simulink model "Hexa_CAD_ANSFT_Sim_V3"  (R2023a)
settings: Solver=ode4  StartTime=0.0  StopTime=30  FixedStep=0.01  RelTol=1e-3
model workspace (MAT data in the model file):
  hover_2m = [0 0 2 0 0 0 0 0 2 0 0 0 ... (36 elements, 6x6)]
  square = [0 0 2.5 0 0 0 0 0 2.5 0 0 0 ... (36 elements, 6x6)]
  tf : Simulink.Parameter (value not decoded)
  tray0 = [0 0 0 0 0 0 0.2 0.15 2 0 0 0 ... (36 elements, 6x6)]
  tray1 = [0 0 0 0 0 0 0 0 2 0 0 0 ... (36 elements, 6x6)]
  tray2 = [0 0 0 0 0 0 2 0 5 0 0 0 ... (36 elements, 6x6)]
  tray3 = [0 0 0 0 0 0 2 0 5 0 0 0 ... (36 elements, 6x6)]
  tray4 = [0 0 0 0 0 0 2 0 5 0.15 0 0 ... (36 elements, 6x6)]
  tray5 = [0 0 0 0 0 0 0 0 5 0.15 0 0 ... (36 elements, 6x6)]
  tray_yaw = [0 0 0 0 0 0 0 0 5 0 0 0 ... (36 elements, 6x6)]
undefined symbols (not defined in the file or in its folder): F, Light, MIL, smiData, X, Y, Z
libraries: sm_lib x168, nesl_utility x33, dspsrcs4 x9, sharedtransform x3, simulink x3, robotcorelib x1, aerolibwind2 x1
(part 3 of 6)

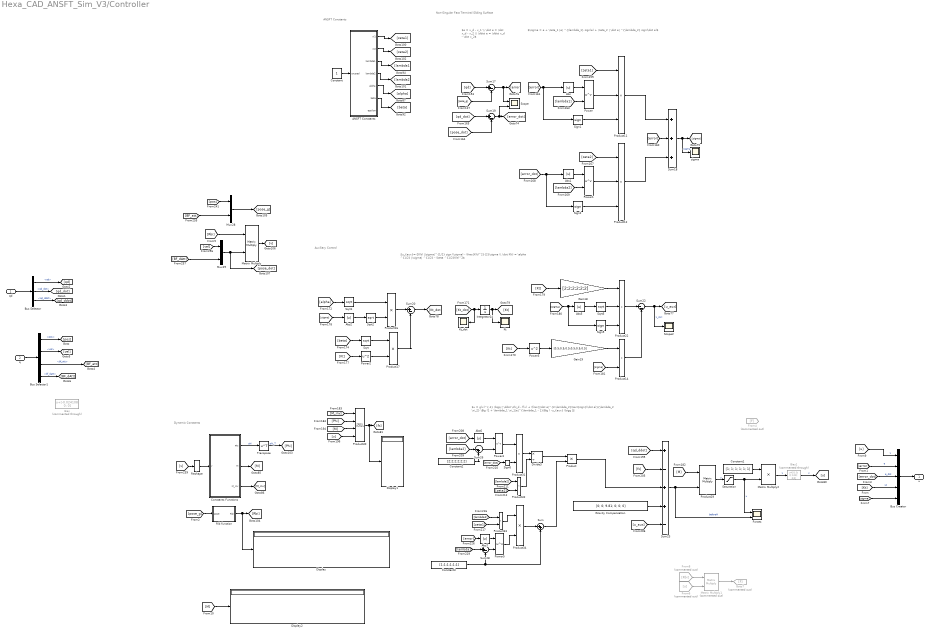
== system Hexa_CAD_ANSFT_Sim_V3/Controller ==
  note: $u = g(x)^{-1} \bigg [ \ddot \chi_d - f(x) + \frac{|\dot e|^{2-\lambda_2}\text{sign}(\dot e)}{\lambda_2 \xi_2} \Big (1 + \lambda_1 \xi_1|e|^{\lambda_1 - 1}\Big ) -u_{aux} \bigg ]$
  note: $e = x_d - x_1 \\ \dot e = \dot x_d - x_2 \\ \ddot e = \ddot x_d - \dot x_2$
  note: Non-Singular Fast Terminal Sliding Surface
  note: $\sigma = e + \zeta_1 |e| ^{\lambda_1} sign(e) + \zeta_2 | \dot e| ^{\lambda_2} sign(\dot e)$
  note: $u_{aux}=-2K(t) |\sigma|^{1/2} sign (\sigma) - \frac{K(t)^2}{2}\sigma \\ \dot K(t) = \alpha ^{1/2} |\sigma| ^{1/2} - \beta ^{1/2}K(t)^2$
  note: Auxiliary Control
  note: ANSFT Constants
  note: Dynamic Constants
  qd : Inport
  q : Inport  Port=2
  ANSFT Constants : MATLAB Function  TreatAsAtomicUnit=on
  Abs{,1..2,5..7} (6 alike) : Abs  SaturateOnIntegerOverflow=off
  Bias : Bias  Commented=through  Bias=[-0.024108; 0; 0]  SaturateOnIntegerOverflow=off
  Bias1 : Bias  Commented=through  Bias=[0; 0; 0; 0.02; 0;0]  SaturateOnIntegerOverflow=off
  Bus Creator : BusCreator  Inputs=5
  Bus Selector : BusSelector  OutputSignals=qd,qd_dot,qd_ddot
  Bus Selector1 : BusSelector  OutputSignals=pos,vel,bf_att,bf_datt
  Constant : Constant
  Constant1 : Constant  Value=[1; 1; 1; 1; 1; 1]
  Constant2 : Constant  Value=[2;2;2;2;2;2]
  Constant3 : Constant  Value=[1;1;1;1;1;1]
  Constants Functions : MATLAB Function  TreatAsAtomicUnit=on
  Display : Display
  Display1 : Display
  Display2 : Display
  Divide3 : Product  Inputs=*/
  Forces : Scope  NumInputPorts=2
  From4 : From  Commented=on  GotoTag=F
  From6 : From  Commented=on  GotoTag=u
  From8 : From  Commented=on  GotoTag=Rbi
  Gain18 : Gain  Gain=[2;2;2;2;2;2]
  Gain19 : Gain  Gain=[0.5;0.5;0.5;0.5;0.5;0.5]
  Goto7 : Goto  Commented=on  GotoTag=F
  Gravity Compensation : Constant  Value=[0; 0; 9.81; 0; 0; 0]
  Integrator14 : Integrator  InitialCondition=[0;0;0;0;0;0]
  Kt : Scope
  Kt_dot : Scope
  Matrix Multiply : Product  Multiplication=Matrix(*)
  Matrix Multiply1 : Product  Commented=on  Multiplication=Matrix(*)
  Matrix Multiply2 : Product
  Mux28 : Mux  Inputs=2
  Mux29 : Mux  Inputs=2
  Power{,1,4..5} (4 alike) : Math  Operator=pow
  Power2 : Math  Operator=square
  Power3 : Math  Operator=square
  Product{,14,16..17,31..34} (8 alike) : Product
  Product11 : Product  Inputs=3
  Product12 : Product  Inputs=3
  Product22 : Product  Inputs=3
  Product29 : Product  Multiplication=Matrix(*)
  Product30 : Product  Inputs=4  Multiplication=Matrix(*)
  Reshape : Reshape  OutputDimensionality=Customize  OutputDimensions=[6,1]
  Rib function : MATLAB Function  TreatAsAtomicUnit=on
  Saturation : Saturate  UpperLimit=[5; 5; 35; 0.2; 0.2; 0.2]  LowerLimit=[-5; -5; 0; -0.2; -0.2; -0.2]
  Scope : Scope  NumInputPorts=2
  Scope2 : Scope
  Sign{1..2,5..6} (4 alike) : Signum
  Sqrt{,1..2,5} (4 alike) : Sqrt
  Sum : Sum  Inputs=|++
  Sum{17,19..20,28} (4 alike) : Sum  Inputs=|+-
  Sum18 : Sum  Inputs=+++
  Sum22 : Sum  Inputs=|--
  Sum23 : Sum  Inputs=+-++-
  Sum26 : Sum  Inputs=|-+
  Transpose : Math  Operator=transpose
  sigma : Scope
  u : Outport
  wires:
  [zeta2] -> Product12/1
  [lambda1] -> Power/2
  Abs1/1 -> Power1/1
  [Kt] -> Power3/1
  [pose_g] -> Sum17/2
  Power5/1 -> Product34/2
  ANSFT Constants/4(lambda2) -> [lambda2]
  [Phi] -> Product30/2
  Product17/1 -> Sum20/2
  [v] -> Product30/4
  Sum20/1 -> [Kt_dot]
  [zeta2] -> Product32/2
  Sum19/1 -> Scope/2, [error_dot]
  Power4/1 -> Product31/1
  [error] -> Abs7/1
  [M_inv] -> Product30/1
  Product11/1 -> Sum18/1
  [lambda2] -> Power1/2
  [error_dot] -> Sign6/1
  [u_aux] -> Sum23/5
  Gain19/1 -> Product14/1
  [Kt] -> Gain18/1
  Sign2/1 -> Product12/3
  Gravity Compensation/1 -> Sum23/4
  ANSFT Constants/6(beta) -> [beta]
  [lambda1] -> Sum28/1
  Product14/1 -> Sum22/2
  Sum28/1 -> Power5/2
  Gain18/1 -> Product22/1
  Product12/1 -> Sum18/3
  [alpha] -> Sqrt1/1
  Product/1 -> Sum23/3
  Power2/1 -> Product17/2
  [M] -> Product29/1
  [beta] -> Sqrt/1
  [sigma] -> Abs2/1
  [fx] -> Sum23/2
  ANSFT Constants/3(lambda1) -> [lambda1]
  [M] -> Product30/3
  Product16/1 -> Sum20/1
  [error_dot] -> Sign2/1, Abs1/1
  Sqrt1/1 -> Product16/1
  Sqrt/1 -> Product17/1
  Abs2/1 -> Sqrt2/1
  [lambda2] -> Sum26/1
  [zeta1] -> Product33/2
  Sign6/1 -> Product31/2
  [qd_ddot] -> Sum23/1
  [error_dot] -> Abs6/1
  [lambda2] -> Product32/1
  Sign5/1 -> Product22/3
  Constant3/1 -> Sum28/2, Sum/2
  [zeta1] -> Product11/1
  ANSFT Constants/1(xi1) -> [zeta1]
  [sigma] -> Sign5/1, Abs5/1
  [error] -> Sum18/2
  Abs7/1 -> Power5/1
  Sum17/1 -> Scope/1, [error]
  Power/1 -> Product11/2
  Constant2/1 -> Sum26/2
  [sigma] -> Product14/2
  ANSFT Constants/5(alpha) -> [alpha]
  [qd_dot] -> Sum19/1
  Product32/1 -> Divide3/2
  [pose_dot] -> Sum19/2
  Sum23/1 -> Forces/2, Product29/2  "beforeM"
  Sum22/1 -> Scope2/1, [u_aux]  "u_aux"
  Abs/1 -> Power/1
  Abs5/1 -> Sqrt5/1
  Product33/1 -> Product34/1
  Product31/1 -> Divide3/1
  [error] -> Sign1/1, Abs/1
  Integrator14/1 -> Kt/1, [Kt]
  [Kt_dot] -> Kt_dot/1, Integrator14/1
  Sqrt5/1 -> Product22/2
  Product22/1 -> Sum22/1
  [Kt] -> Power2/1
  Sum18/1 -> sigma/1, [sigma]  "sigma"
  Power1/1 -> Product12/2
  [qd] -> Sum17/1
  Abs6/1 -> Power4/1
  Sum26/1 -> Power4/2
  ANSFT Constants/2(xi2) -> [zeta2]
  Divide3/1 -> Product/1
  Sqrt2/1 -> Product16/2
  Product30/1 -> Display1/1, [fx]
  [lambda1] -> Product33/1
  Constant/1 -> ANSFT Constants/1(unused)
  Sign1/1 -> Product11/3
  Power3/1 -> Gain19/1
  qd/1 -> Bus Selector/1
  Bus Selector/2 -> [qd_dot]  "<qd_dot>"
  Bus Selector/1 -> [qd]  "<qd>"
  Bus Selector/3 -> [qd_ddot]  "<qd_ddot>"
  Reshape/1 -> Constants Functions/1(v)
  Constants Functions/1(Phi) -> Transpose/1  "phi"
  Constants Functions/2(M) -> [M]
  Rib function/1(Rbi) -> Display/1, [Rbi]
  [v] -> Reshape/1
  Constants Functions/3(M_inv) -> [M_inv]
  [pose_g] -> Rib function/1(pose)
  Transpose/1 -> [Phi]  "phi_T"
  Mux28/1 -> [pose_g]
  Mux29/1 -> [pose_dot], Matrix Multiply/2
  [BF_dAtt] -> Mux29/2
  Matrix Multiply/1 -> [v]
  [Rbi] -> Matrix Multiply/1
  [pos] -> Mux28/1
  [BF_att] -> Mux28/2
  [vel] -> Mux29/1
  Bus Creator/1 -> u/1
  [error_dot] -> Bus Creator/3  "e_dot"
  [sigma] -> Bus Creator/5
  [Kt] -> Bus Creator/4  "kt"
  [error] -> Bus Creator/2  "e"
  q/1 -> Bus Selector1/1
  Bus Selector1/1 -> [pos]  "<pos>"
  Bus Selector1/3 -> [BF_att]  "<bf_att>"
  Bus Selector1/2 -> [vel]  "<vel>"
  Bus Selector1/4 -> [BF_dAtt]  "<bf_datt>"
  Product34/1 -> Sum/1
  Sum/1 -> Product/2
  Product29/1 -> Saturation/1  "u"
  From6/1 -> Matrix Multiply1/2
  From8/1 -> Matrix Multiply1/1
  Matrix Multiply1/1 -> Goto7/1
  [u] -> Bus Creator/1  "u"
  Saturation/1 -> Matrix Multiply2/2, Forces/1  "u"
  [M] -> Display2/1
  Matrix Multiply2/1 -> Bias1/1  "u"
  Constant1/1 -> Matrix Multiply2/1
  Bias1/1 -> [u]  "u"

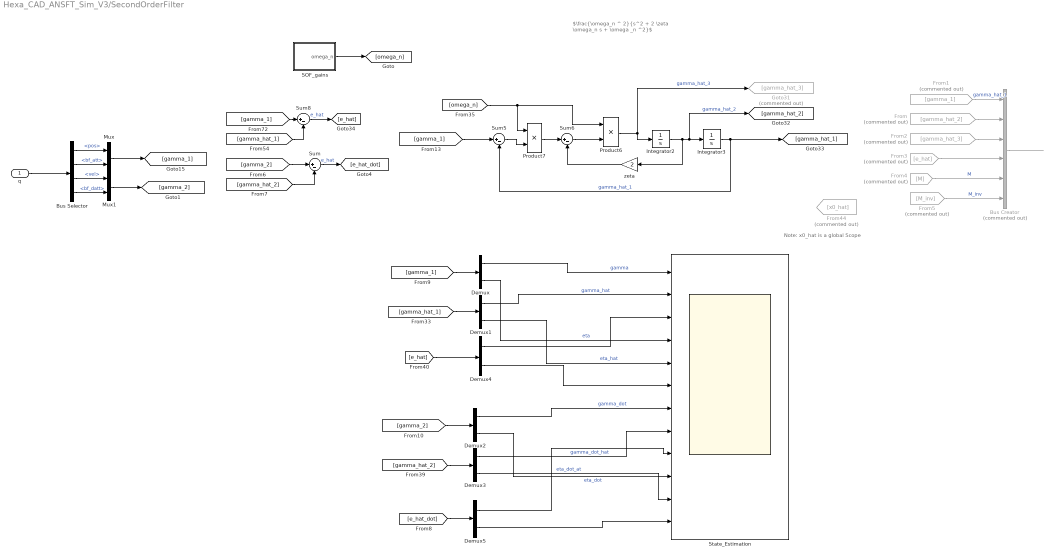
== system Hexa_CAD_ANSFT_Sim_V3/SecondOrderFilter ==
  note: Note: x0_hat is a global Scope
  note: $\frac{\omega_n ^ 2}{s^2 + 2 \zeta \omega_n s + \omega _n ^2}$
  q : Inport
  Bus Creator : BusCreator  Commented=on  Inputs=6
  Bus Selector : BusSelector  OutputSignals=pos,bf_att,vel,bf_datt
  Demux{,1..5} (6 alike) : Demux  Outputs=2
  From : From  Commented=on  GotoTag=gamma_hat_2
  From1 : From  Commented=on  GotoTag=gamma_1
  From2 : From  Commented=on  GotoTag=gamma_hat_3
  From3 : From  Commented=on  GotoTag=e_hat
  From4 : From  Commented=on  GotoTag=M
  From44 : From  Commented=on  GotoTag=x0_hat  TagVisibility=global
  From5 : From  Commented=on  GotoTag=M_inv
  Goto31 : Goto  Commented=on  GotoTag=gamma_hat_3
  Integrator2 : Integrator
  Integrator3 : Integrator
  Mux : Mux  Inputs=2
  Mux1 : Mux  Inputs=2
  Product6 : Product
  Product7 : Product
  SOF_gains : MATLAB Function  TreatAsAtomicUnit=on
  State_Estimation : Scope  NumInputPorts=12
  Sum{,5..6,8} (4 alike) : Sum  Inputs=|+-
  zeta : Gain  Gain=2
  wires:
  [gamma_1] -> Sum5/1
  Integrator3/1 -> Sum5/2, [gamma_hat_1]  "gamma_hat_1"
  zeta/1 -> Sum6/2
  Sum8/1 -> [e_hat]  "e_hat"
  [omega_n] -> Product7/1, Product6/1
  Sum6/1 -> Product6/2
  Product6/1 -> Integrator2/1, Goto31/1  "gamma_hat_3"
  Integrator2/1 -> zeta/1, [gamma_hat_2], Integrator3/1  "gamma_hat_2"
  [gamma_1] -> Sum8/1
  Sum5/1 -> Product7/2
  Product7/1 -> Sum6/1
  [gamma_hat_1] -> Sum8/2
  q/1 -> Bus Selector/1
  SOF_gains/1(omega_n) -> [omega_n]
  From1/1 -> Bus Creator/1  "gamma_hat_1"
  From/1 -> Bus Creator/2
  From2/1 -> Bus Creator/3
  From3/1 -> Bus Creator/4
  Bus Creator/1 -> ?
  From4/1 -> Bus Creator/5  "M"
  From5/1 -> Bus Creator/6  "M_inv"
  [gamma_2] -> Sum/1
  [gamma_hat_2] -> Sum/2
  Sum/1 -> [e_hat_dot]  "e_hat"
  Demux5/1 -> State_Estimation/9
  [gamma_hat_2] -> Demux3/1
  Demux1/1 -> State_Estimation/2  "gamma_hat"
  Demux2/2 -> State_Estimation/10  "eta_dot"
  Demux/2 -> State_Estimation/4  "eta"
  [gamma_hat_1] -> Demux1/1
  Demux5/2 -> State_Estimation/12
  Demux3/2 -> State_Estimation/11  "eta_dot_at"
  Demux1/2 -> State_Estimation/5  "eta_hat"
  [gamma_2] -> Demux2/1
  Demux3/1 -> State_Estimation/8  "gamma_dot_hat"
  Demux2/1 -> State_Estimation/7  "gamma_dot"
  [gamma_1] -> Demux/1
  [e_hat] -> Demux4/1
  Demux/1 -> State_Estimation/1  "gamma"
  Demux4/1 -> State_Estimation/3
  [e_hat_dot] -> Demux5/1
  Demux4/2 -> State_Estimation/6
  Bus Selector/1 -> Mux/1  "<pos>"
  Bus Selector/2 -> Mux/2  "<bf_att>"
  Mux/1 -> [gamma_1]
  Bus Selector/3 -> Mux1/1  "<vel>"
  Mux1/1 -> [gamma_2]
  Bus Selector/4 -> Mux1/2  "<bf_datt>"

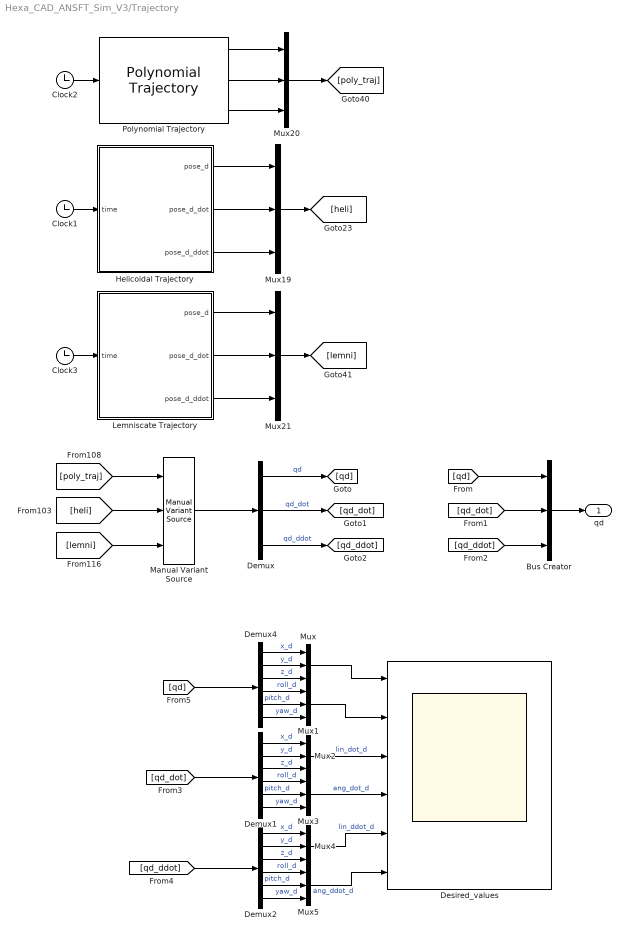
== system Hexa_CAD_ANSFT_Sim_V3/Trajectory ==
  Bus Creator : BusCreator  Inputs=3
  Clock1 : Clock
  Clock2 : Clock
  Clock3 : Clock
  Demux : Demux  Outputs=3
  Demux1 : Demux  Outputs=6
  Demux2 : Demux  Outputs=6
  Demux4 : Demux  Outputs=6
  Desired_values : Scope  NumInputPorts=6
  Helicoidal Trajectory : MATLAB Function  TreatAsAtomicUnit=on
  Lemniscate Trajectory : MATLAB Function  TreatAsAtomicUnit=on
  Manual Variant Source : simulink/Signal Routing/Manual Variant Source  NumChoices=3  LabelModeActiveChoice=V_1
  Mux{,1..5,19..21} (9 alike) : Mux  Inputs=3
  Polynomial Trajectory : robotcorelib/Polynomial Trajectory  WaypointSource=Internal  Waypoints=tray1  TimePoints=[ 0, 12, 24, 36, 48, tf ]  TimeInterval=[ 1, 4 ]  Method=Cubic Polynomial  ParameterSource=Internal  VelocityBoundaryCondition=zeros( 6, 6 )  AccelerationBoundaryCondition=zeros( 2, 5 )  SimulateUsing=Interpreted execution
  qd : Outport
  wires:
  Polynomial Trajectory/2 -> Mux20/2
  Polynomial Trajectory/1 -> Mux20/1
  Lemniscate Trajectory/1(pose_d) -> Mux21/1
  Clock3/1 -> Lemniscate Trajectory/1(time)
  Polynomial Trajectory/3 -> Mux20/3
  Clock2/1 -> Polynomial Trajectory/1
  Helicoidal Trajectory/1(pose_d) -> Mux19/1
  Lemniscate Trajectory/3(pose_d_ddot) -> Mux21/3
  Mux21/1 -> [lemni]
  Mux19/1 -> [heli]
  Helicoidal Trajectory/2(pose_d_dot) -> Mux19/2
  Clock1/1 -> Helicoidal Trajectory/1(time)
  Mux20/1 -> [poly_traj]
  Helicoidal Trajectory/3(pose_d_ddot) -> Mux19/3
  Lemniscate Trajectory/2(pose_d_dot) -> Mux21/2
  Demux/3 -> [qd_ddot]  "qd_ddot"
  Demux/1 -> [qd]  "qd"
  Demux4/1 -> Mux/1  "x_d"
  Demux2/5 -> Mux5/2  "pitch_d"
  Demux/2 -> [qd_dot]  "qd_dot"
  [qd_ddot] -> Bus Creator/3
  Demux1/5 -> Mux3/2  "pitch_d"
  Demux1/3 -> Mux2/3  "z_d"
  Demux4/6 -> Mux1/3  "yaw_d"
  [qd_dot] -> Demux1/1
  [heli] -> Manual Variant Source/2
  Demux1/2 -> Mux2/2  "y_d"
  Mux1/1 -> Desired_values/2
  Demux4/3 -> Mux/3  "z_d"
  Demux4/2 -> Mux/2  "y_d"
  Demux1/1 -> Mux2/1  "x_d"
  [qd_ddot] -> Demux2/1
  Mux2/1 -> Desired_values/3  "lin_dot_d"
  Demux4/5 -> Mux1/2  "pitch_d"
  Mux5/1 -> Desired_values/6  "ang_ddot_d"
  Demux2/3 -> Mux4/3  "z_d"
  [qd] -> Demux4/1
  Mux3/1 -> Desired_values/4  "ang_dot_d"
  [qd_dot] -> Bus Creator/2
  Demux4/4 -> Mux1/1  "roll_d"
  Mux/1 -> Desired_values/1
  Demux1/4 -> Mux3/1  "roll_d"
  [lemni] -> Manual Variant Source/3
  Demux2/1 -> Mux4/1  "x_d"
  Demux1/6 -> Mux3/3  "yaw_d"
  Mux4/1 -> Desired_values/5  "lin_ddot_d"
  Bus Creator/1 -> qd/1
  Demux2/4 -> Mux5/1  "roll_d"
  [qd] -> Bus Creator/1
  [poly_traj] -> Manual Variant Source/1
  Manual Variant Source/1 -> Demux/1
  Demux2/6 -> Mux5/3  "yaw_d"
  Demux2/2 -> Mux4/2  "y_d"

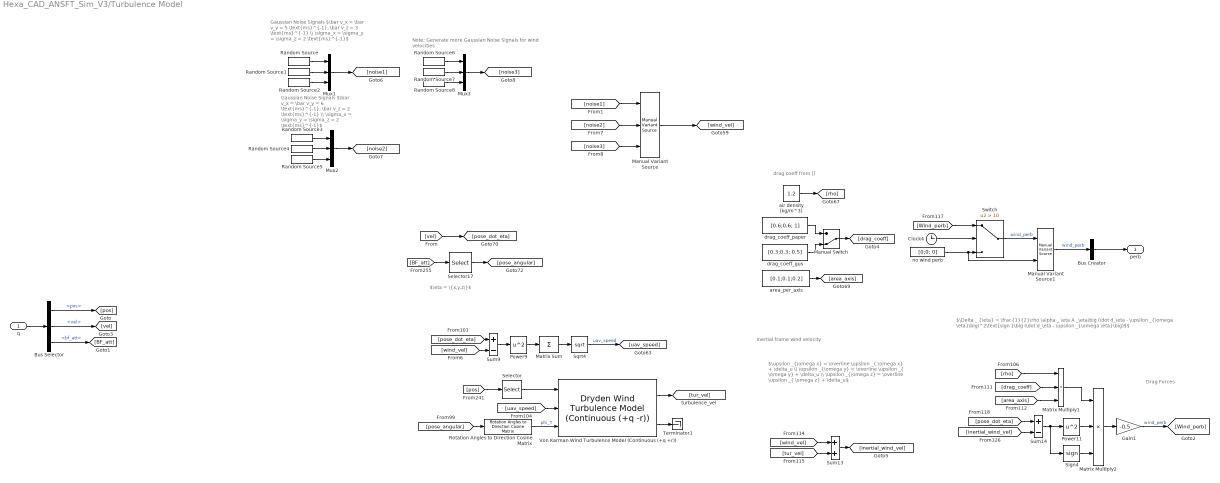
== system Hexa_CAD_ANSFT_Sim_V3/Turbulence Model ==
  note: Note: Generate more Gaussian Noise Signals
      | for wind velocities
  note: $\Delta _ {\eta} = \frac{1}{2}\rho \alpha _ \eta A _\eta\big (\dot d_\eta - \upsilon _{\omega \eta}\big)^2\text{sign }\big (\dot d_\eta - \upsilon _{\omega \eta}\big)$$
  note: $\upsilon _{\omega x} = \overline \upsilon _{ \omega x} + \delta_u \\ \upsilon _{\omega y} = \overline \upsilon _{ \omega y} + \delta_u \\ \upsilon _{\omega z} = \overline \upsilon _{ \omega z} + \delta_u$
  note: drag coeff from []
  note: Drag Forces
  note: Inertial frame wind velocity
  note: $\eta = \{x,y,z\}$
  note: Gaussian Noise Signals
      | $\bar v_x = \bar v_y = 6 \text{ms}^{-1}, \bar v_z = 2 \text{ms}^{-1} \\ \sigma_x = \sigma_y = \sigma_z = 2 \text{ms}^{-1}$
  note: Gaussian Noise Signals
      | $\bar v_x = \bar v_y = 5 \text{ms}^{-1}, \bar v_z = 3 \text{ms}^{-1} \\ \sigma_x = \sigma_y = \sigma_z = 2 \text{ms}^{-1}$
  q : Inport
  Bus Creator : BusCreator  Inputs=1
  Bus Selector : BusSelector  OutputSignals=pos,vel,bf_att
  Clock4 : Clock
  Gain1 : Gain  Gain=-0.5
  Manual Variant Source : simulink/Signal Routing/Manual Variant Source  NumChoices=3  LabelModeActiveChoice=V_1
  Manual Variant Source1 : simulink/Signal Routing/Manual Variant Source  NumChoices=2  LabelModeActiveChoice=V_1
  Manual Switch : ManualSwitch  CurrentSetting=0
  Matrix Sum : Sum  Inputs=+
  Matrix Multiply1 : Product  Inputs=3
  Matrix Multiply2 : Product  Inputs=3
  Mux1 : Mux  Inputs=3
  Mux2 : Mux  Inputs=3
  Mux3 : Mux  Inputs=3
  Power11 : Math  Operator=square
  Power9 : Math  Operator=square
  Random Source : dspsrcs4/Random Source  SrcType=Gaussian  NormMethod=Ziggurat  CltLength=12  MinVal=0  MaxVal=1  MeanVal=5  VarVal=2  RepMode=Not repeatable  rawSeed=1  IsInherit=off  SampMode=Discrete  SampTime=1  SampFrame=1  DataType=Double  OutComplex=Real  OutputFrames=off
  Random Source1 : dspsrcs4/Random Source  SrcType=Gaussian  NormMethod=Ziggurat  CltLength=12  MinVal=0  MaxVal=1  MeanVal=5  VarVal=2  RepMode=Not repeatable  rawSeed=1  IsInherit=off  SampMode=Discrete  SampTime=1  SampFrame=1  DataType=Double  OutComplex=Real  OutputFrames=off
  Random Source2 : dspsrcs4/Random Source  SrcType=Gaussian  NormMethod=Ziggurat  CltLength=12  MinVal=0  MaxVal=1  MeanVal=3  VarVal=2  RepMode=Not repeatable  rawSeed=1  IsInherit=off  SampMode=Discrete  SampTime=1  SampFrame=1  DataType=Double  OutComplex=Real  OutputFrames=off
  Random Source{3..4,6..7} (4 alike) : dspsrcs4/Random Source  SrcType=Gaussian  NormMethod=Ziggurat  CltLength=12  MinVal=0  MaxVal=1  MeanVal=6  VarVal=2  RepMode=Not repeatable  rawSeed=1  IsInherit=off  SampMode=Discrete  SampTime=1  SampFrame=1  DataType=Double  OutComplex=Real  OutputFrames=off
  Random Source5 : dspsrcs4/Random Source  SrcType=Gaussian  NormMethod=Ziggurat  CltLength=12  MinVal=0  MaxVal=1  MeanVal=2  VarVal=2  RepMode=Not repeatable  rawSeed=1  IsInherit=off  SampMode=Discrete  SampTime=1  SampFrame=1  DataType=Double  OutComplex=Real  OutputFrames=off
  Random Source8 : dspsrcs4/Random Source  SrcType=Gaussian  NormMethod=Ziggurat  CltLength=12  MinVal=0  MaxVal=1  MeanVal=2  VarVal=2  RepMode=Not repeatable  rawSeed=1  IsInherit=off  SampMode=Discrete  SampTime=1  SampFrame=1  DataType=Double  OutComplex=Real  OutputFrames=off
  Rotation Angles to Direction Cosine Matrix : sharedtransform/Rotation Angles to Direction Cosine Matrix  rotationOrder=XYZ  aMode=aMode
  Selector : Selector  InputPortWidth=3  IndexOptions=Index vector (dialog)  Indices=[3]  OutputSizes=1
  Selector17 : Selector  InputPortWidth=3  IndexOptions=Index vector (dialog)  Indices=[3 2 1]  OutputSizes=1
  Sign4 : Signum
  Sqrt4 : Sqrt
  Sum13 : Sum
  Sum14 : Sum  Inputs=+-
  Sum9 : Sum  Inputs=+-
  Switch : Switch  Criteria=u2 > Threshold  Threshold=10  SaturateOnIntegerOverflow=off  InputSameDT=off
  Terminator1 : Terminator
  Von Karman Wind Turbulence Model (Continuous (+q +r)) : aerolibwind2/Dryden Wind Turbulence Model  (Continuous (+q -r))  units=Metric (MKS)  spec=MIL-F-8785C  model=Continuous Von Karman (+q -r)  W20=15  Wdeg=0  TurbProb=10^-2 - Light  L_high=762  Wingspan=10  ts=0.1  Seed=[23341 23342 23343 23344]  T_on=on
      settings: LibrarySourceBlock=|
      | aerolibwind2/Von Karman Wind Turbulence Model
      | (Continuous (+q +r))
  air density [kg/m^3] : Constant  Value=1.2
  area_per_axis : Constant  Value=[0.1;0.1;0.2]
  drag_coeff_gus : Constant  Value=[0.3;0.3; 0.5]
  drag_coeff_paper : Constant  Value=[0.6;0.6; 1]
  no wind perb : Constant  Value=[0;0; 0]
  perb : Outport
  wires:
  [rho] -> Matrix Multiply1/1
  [drag_coeff] -> Matrix Multiply1/2
  Von Karman Wind Turbulence Model (Continuous (+q +r))/2 -> Terminator1/1
  area_per_axis/1 -> [area_axis]
  [pose_dot_eta] -> Sum14/1
  Von Karman Wind Turbulence Model (Continuous (+q +r))/1 -> [tur_vel]
  [wind_vel] -> Sum9/2
  Selector17/1 -> [pose_angular]
  Matrix Multiply1/1 -> Matrix Multiply2/1
  Sign4/1 -> Matrix Multiply2/3
  [uav_speed] -> Von Karman Wind Turbulence Model (Continuous (+q +r))/2
  Power9/1 -> Matrix Sum/1
  Sqrt4/1 -> [uav_speed]  "uav_speed"
  Gain1/1 -> [Wind_perb]  "wind_perb"
  Sum9/1 -> Power9/1
  air density [kg/m^3]/1 -> [rho]
  Clock4/1 -> Switch/2
  [pose_dot_eta] -> Sum9/1
  Rotation Angles to Direction Cosine Matrix/1 -> Von Karman Wind Turbulence Model (Continuous (+q +r))/3  "phi_T"
  [tur_vel] -> Sum13/2
  Sum14/1 -> Sign4/1, Power11/1
  no wind perb/1 -> Manual Variant Source1/2, Switch/3
  drag_coeff_gus/1 -> Manual Switch/2
  Switch/1 -> Manual Variant Source1/1  "wind_perb"
  [area_axis] -> Matrix Multiply1/3
  Manual Switch/1 -> [drag_coeff]
  Selector/1 -> Von Karman Wind Turbulence Model (Continuous (+q +r))/1
  [pose_angular] -> Rotation Angles to Direction Cosine Matrix/1
  [inertial_wind_vel] -> Sum14/2
  Matrix Multiply2/1 -> Gain1/1
  drag_coeff_paper/1 -> Manual Switch/1
  Power11/1 -> Matrix Multiply2/2
  Matrix Sum/1 -> Sqrt4/1
  Sum13/1 -> [inertial_wind_vel]
  [Wind_perb] -> Switch/1
  [wind_vel] -> Sum13/1
  Bus Creator/1 -> perb/1
  [BF_att] -> Selector17/1
  [pos] -> Selector/1
  q/1 -> Bus Selector/1
  Bus Selector/1 -> [pos]  "<pos>"
  Bus Selector/3 -> [BF_att]  "<bf_att>"
  Bus Selector/2 -> [vel]  "<vel>"
  [vel] -> [pose_dot_eta]
  Mux2/1 -> [noise2]
  Random Source5/1 -> Mux2/3
  Random Source/1 -> Mux1/1
  Mux1/1 -> [noise1]
  Random Source2/1 -> Mux1/3
  Random Source4/1 -> Mux2/2
  Random Source3/1 -> Mux2/1
  [noise2] -> Manual Variant Source/2
  Manual Variant Source/1 -> [wind_vel]
  Random Source1/1 -> Mux1/2
  [noise1] -> Manual Variant Source/1
  [noise3] -> Manual Variant Source/3
  Mux3/1 -> [noise3]
  Random Source7/1 -> Mux3/2
  Random Source6/1 -> Mux3/1
  Random Source8/1 -> Mux3/3
  Manual Variant Source1/1 -> Bus Creator/1  "wind_perb"

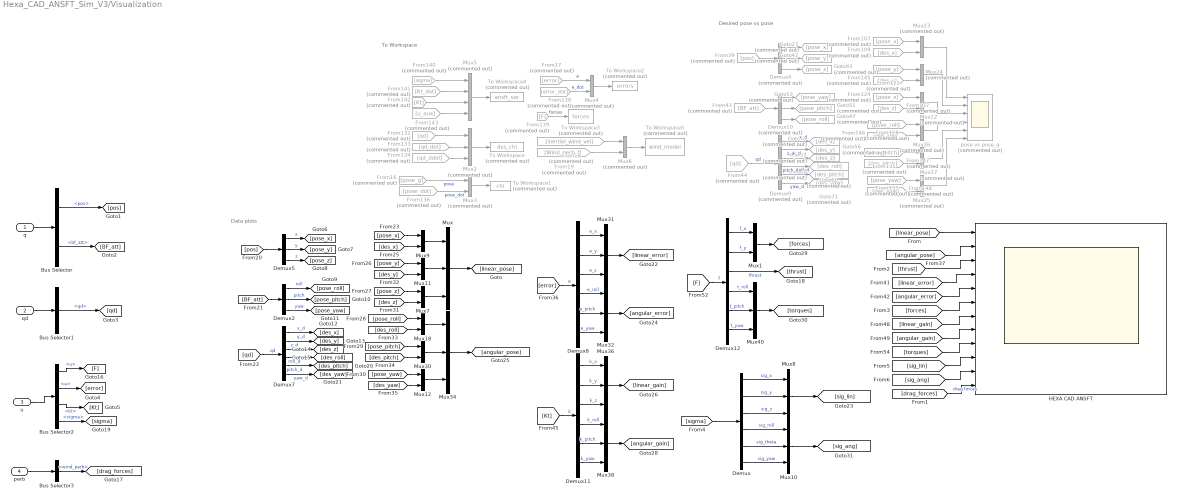
== system Hexa_CAD_ANSFT_Sim_V3/Visualization ==
  note: Desired pose vs pose
  note: Data plots
  note: To Workspace
  q : Inport
  qd : Inport  Port=2
  u : Inport  Port=3
  perb : Inport  Port=4
  Bus Selector : BusSelector  OutputSignals=pos,bf_att
  Bus Selector1 : BusSelector  OutputSignals=qd
  Bus Selector2 : BusSelector  OutputSignals=u,e,kt,sigma
  Bus Selector3 : BusSelector  OutputSignals=wind_perb
  Demux{,7..8,11..12} (5 alike) : Demux  Outputs=6
  Demux10 : Demux  Commented=on  Outputs=3
  Demux2 : Demux  Outputs=3
  Demux4 : Demux  Commented=on  Outputs=3
  Demux5 : Demux  Outputs=3
  Demux9 : Demux  Commented=on  Outputs=6
  From107 : From  Commented=on  GotoTag=pose_x
  From109 : From  Commented=on  GotoTag=des_x
  From122 : From  Commented=on  GotoTag=pose_y
  From124 : From  Commented=on  GotoTag=pose_z
  From128 : From  Commented=on  GotoTag=pose_roll
  From131 : From  Commented=on  GotoTag=pose_pitch
  From132 : From  Commented=on  GotoTag=qd
  From133 : From  Commented=on  GotoTag=qd_dot
  From134 : From  Commented=on  GotoTag=qd_ddot
  From135 : From  Commented=on  GotoTag=pose_yaw
  From136 : From  Commented=on  GotoTag=pose_dot
  From137 : From  Commented=on  GotoTag=des_z
  From138 : From  Commented=on  GotoTag=error_dot
  From139 : From  Commented=on  GotoTag=F
  From140 : From  Commented=on  GotoTag=sigma
  From141 : From  Commented=on  GotoTag=Kt_dot
  From142 : From  Commented=on  GotoTag=Kt
  From143 : From  Commented=on  GotoTag=u_aux
  From145 : From  Commented=on  GotoTag=des_y
  From146 : From  Commented=on  GotoTag=des_roll
  From147 : From  Commented=on  GotoTag=des_pitch
  From148 : From  Commented=on  GotoTag=des_yaw
  From16 : From  Commented=on  GotoTag=pose_g
  From17 : From  Commented=on  GotoTag=error
  From18 : From  Commented=on  GotoTag=inertial_wind_vel
  From19 : From  Commented=on  GotoTag=Wind_perb_f  TagVisibility=global
  From39 : From  Commented=on  GotoTag=pos
  From43 : From  Commented=on  GotoTag=BF_att
  From44 : From  Commented=on  GotoTag=qd
  Goto27 : Goto  Commented=on  GotoTag=pose_x
  Goto42 : Goto  Commented=on  GotoTag=pose_y
  Goto43 : Goto  Commented=on  GotoTag=pose_z
  Goto47 : Goto  Commented=on  GotoTag=pose_roll
  Goto51 : Goto  Commented=on  GotoTag=pose_pitch
  Goto53 : Goto  Commented=on  GotoTag=pose_yaw
  Goto55 : Goto  Commented=on  GotoTag=des_x
  Goto56 : Goto  Commented=on  GotoTag=des_y
  Goto57 : Goto  Commented=on  GotoTag=des_z
  Goto60 : Goto  Commented=on  GotoTag=des_roll
  Goto68 : Goto  Commented=on  GotoTag=des_pitch
  Goto71 : Goto  Commented=on  GotoTag=des_yaw
  HEXA CAD ANSFT : Scope  NumInputPorts=12
  Mux{,8,10,31..32,34,36,38,40} (9 alike) : Mux  Inputs=3
  Mux{1,7,9,11..12,18,30} (7 alike) : Mux  Inputs=2
  Mux2 : Mux  Commented=on  Inputs=3
  Mux{3..4,6,22..27} (9 alike) : Mux  Commented=on  Inputs=2
  Mux5 : Mux  Commented=on
  To Workspace : ToWorkspace  Commented=on  VariableName=des_chi  SaveFormat=Structure With Time  SampleTime=-1
  To Workspace1 : ToWorkspace  Commented=on  VariableName=chi  SaveFormat=Structure With Time  SampleTime=-1
  To Workspace2 : ToWorkspace  Commented=on  VariableName=errors  SaveFormat=Structure With Time  SampleTime=-1
  To Workspace3 : ToWorkspace  Commented=on  VariableName=forces  SaveFormat=Structure With Time  SampleTime=-1
  To Workspace4 : ToWorkspace  Commented=on  VariableName=ansft_var  SaveFormat=Structure With Time  SampleTime=-1
  To Workspace5 : ToWorkspace  Commented=on  VariableName=wind_model  SaveFormat=Structure With Time  SampleTime=-1
  pose vs pose_q : Scope  Commented=on  NumInputPorts=6
  wires:
  Mux/1 -> [linear_pose]
  Mux6/1 -> To Workspace5/1
  Mux9/1 -> Mux/1
  From128/1 -> Mux26/1
  Demux4/1 -> Goto27/1
  Demux7/5 -> [des_pitch]  "pitch_d"
  From135/1 -> Mux25/1
  [linear_error] -> HEXA CAD ANSFT/4
  [angular_error] -> HEXA CAD ANSFT/5
  From132/1 -> Mux2/1
  Mux11/1 -> Mux/2
  Demux11/2 -> Mux36/2  "k_y"
  Demux4/3 -> Goto43/1
  Demux5/1 -> [pose_x]  "x"
  Demux10/1 -> Goto53/1
  Demux12/6 -> Mux40/3  "t_yaw"
  Demux12/4 -> Mux40/1  "t_roll"
  Mux40/1 -> [torques]
  Mux1/1 -> [forces]
  Demux10/3 -> Goto47/1
  Mux3/1 -> To Workspace1/1
  Demux5/3 -> [pose_z]  "z"
  Demux11/1 -> Mux36/1  "k_x"
  Demux8/6 -> Mux32/3  "e_yaw"
  From148/1 -> Mux25/2
  Demux11/4 -> Mux38/1  "k_roll"
  Demux9/6 -> Goto71/1  "yaw_d"
  [BF_att] -> Demux2/1
  Mux31/1 -> [linear_error]
  Mux23/1 -> pose vs pose_q/1
  Demux9/2 -> Goto56/1  "y_d"
  Demux7/2 -> [des_y]  "y_d"
  Demux5/2 -> [pose_y]  "y"
  From16/1 -> Mux3/1  "pose"
  [pose_pitch] -> Mux30/1
  [pose_y] -> Mux11/1
  Demux8/3 -> Mux31/3  "e_z"
  From44/1 -> Demux9/1  "qd"
  Demux7/3 -> [des_z]  "z_d"
  Demux12/2 -> Mux1/2  "f_y"
  [angular_gain] -> HEXA CAD ANSFT/8
  [error] -> Demux8/1  "e"
  From133/1 -> Mux2/2
  [des_pitch] -> Mux30/2
  [F] -> Demux12/1  "f"
  Mux5/1 -> To Workspace4/1
  [linear_gain] -> HEXA CAD ANSFT/7
  Mux2/1 -> To Workspace/1
  [des_roll] -> Mux18/2
  From43/1 -> Demux10/1
  Mux22/1 -> pose vs pose_q/3
  Mux26/1 -> pose vs pose_q/4
  Mux24/1 -> pose vs pose_q/2
  Demux12/1 -> Mux1/1  "f_x"
  From109/1 -> Mux23/2
  Demux7/4 -> [des_roll]  "roll_d"
  Demux9/4 -> Goto60/1  "roll_d"
  Demux12/3 -> [thrust]  "thrust"
  From122/1 -> Mux24/1
  Mux36/1 -> [linear_gain]
  [des_yaw] -> Mux12/2
  Demux11/6 -> Mux38/3  "k_yaw"
  From139/1 -> To Workspace3/1  "forces"
  [angular_pose] -> HEXA CAD ANSFT/2
  Demux9/3 -> Goto57/1  "z_d"
  Demux8/1 -> Mux31/1  "e_x"
  From124/1 -> Mux22/1
  Demux7/1 -> [des_x]  "x_d"
  From138/1 -> Mux4/2  "e_dot"
  [pose_yaw] -> Mux12/1
  From39/1 -> Demux4/1
  From137/1 -> Mux22/2
  Mux12/1 -> Mux34/3
  From131/1 -> Mux27/1
  Demux12/5 -> Mux40/2  "t_pitch"
  [des_x] -> Mux9/2
  Demux8/4 -> Mux32/1  "e_roll"
  [linear_pose] -> HEXA CAD ANSFT/1
  Demux9/1 -> Goto55/1  "x_d"
  [pos] -> Demux5/1
  From18/1 -> Mux6/1
  From141/1 -> Mux5/2
  Mux7/1 -> Mux/3
  From145/1 -> Mux24/2
  Demux9/5 -> Goto68/1  "pitch_d"
  From17/1 -> Mux4/1  "e"
  Demux8/5 -> Mux32/2  "e_pitch"
  Mux34/1 -> [angular_pose]
  [pose_x] -> Mux9/1
  Demux10/2 -> Goto51/1
  [pose_roll] -> Mux18/1
  [pose_z] -> Mux7/1
  Mux30/1 -> Mux34/2
  [des_y] -> Mux11/2
  Demux11/3 -> Mux36/3  "k_z"
  Demux7/6 -> [des_yaw]  "yaw_d"
  Mux4/1 -> To Workspace2/1
  From19/1 -> Mux6/2
  From134/1 -> Mux2/3
  Mux38/1 -> [angular_gain]
  Mux18/1 -> Mux34/1
  Demux11/5 -> Mux38/2  "k_pitch"
  Demux4/2 -> Goto42/1
  [Kt] -> Demux11/1  "k"
  Mux32/1 -> [angular_error]
  [qd] -> Demux7/1  "qd"
  Demux8/2 -> Mux31/2  "e_y"
  From143/1 -> Mux5/4
  From146/1 -> Mux26/2
  Mux27/1 -> pose vs pose_q/5
  [des_z] -> Mux7/2
  From147/1 -> Mux27/2
  From142/1 -> Mux5/3
  From140/1 -> Mux5/1
  From136/1 -> Mux3/2  "pose_dot"
  From107/1 -> Mux23/1
  Mux25/1 -> pose vs pose_q/6
  q/1 -> Bus Selector/1
  Bus Selector/1 -> [pos]  "<pos>"
  Bus Selector/2 -> [BF_att]  "<bf_att>"
  qd/1 -> Bus Selector1/1
  Bus Selector1/1 -> [qd]  "<qd>"
  u/1 -> Bus Selector2/1
  Bus Selector2/1 -> [F]  "<u>"
  Bus Selector2/2 -> [error]  "<e>"
  Bus Selector2/3 -> [Kt]  "<kt>"
  perb/1 -> Bus Selector3/1
  Bus Selector3/1 -> [drag_forces]  "<wind_perb>"
  [thrust] -> HEXA CAD ANSFT/3
  [forces] -> HEXA CAD ANSFT/6
  [torques] -> HEXA CAD ANSFT/9
  [drag_forces] -> HEXA CAD ANSFT/12  "drag forces"
  Bus Selector2/4 -> [sigma]  "<sigma>"
  Demux/6 -> Mux10/3  "sig_yaw"
  Demux/5 -> Mux10/2  "sig_theta"
  Demux/3 -> Mux8/3  "sig_z"
  Demux/1 -> Mux8/1  "sig_x"
  Demux/4 -> Mux10/1  "sig_roll"
  Mux10/1 -> [sig_ang]
  Mux8/1 -> [sig_lin]
  [sigma] -> Demux/1
  Demux/2 -> Mux8/2  "sig_y"
  [sig_lin] -> HEXA CAD ANSFT/10
  [sig_ang] -> HEXA CAD ANSFT/11
  Demux2/2 -> [pose_pitch]  "pitch"
  Demux2/3 -> [pose_yaw]  "yaw"
  Demux2/1 -> [pose_roll]  "roll"

== system Hexa_CAD_ANSFT_Sim_V3/6DoF_Dynamics/APC_8X3_8_Slow_Flyer_1_RIGID ==
  ReferenceFrame : sm_lib/Frames and Transforms/Reference Frame
  Solid : sm_lib/Body Elements/File Solid  ExtGeomFileName=APC 8X3.8 Slow Flyer_Valor predeterminado_sldprt.STEP  UnitType=FromFile  ExtGeomFileUnits=m  StepReaderType=HEX  ExportConvexHullGeometry=off  InertiaType=Custom  Mass=smiData.Solid(8).mass  MassUnits=kg  CenterOfMass=smiData.Solid(8).CoM  CenterOfMassUnits=mm  MomentsOfInertia=smiData.Solid(8).MoI  MomentsOfInertiaUnits=kg*mm^2  ProductsOfInertia=smiData.Solid(8).PoI  ProductsOfInertiaUnits=kg*mm^2  BasedOnType=DensityFromFile  Density=1000  DensityUnits=kg/m^3  DoExposeReferenceFrame=on  SerializedFrames=<Frames/>  GraphicType=FromGeometry  MarkerShape=Sphere  MarkerSize=10  GraphicVisPropType=SimpleVisualProperties  GraphicDiffuseColor=smiData.Solid(8).color  GraphicSpecularColor=[0.5 0.5 0.5 1.0]  GraphicAmbientColor=[0.15 0.15 0.15 1.0]  GraphicEmissiveColor=[0.0 0.0 0.0 1.0]  GraphicShininess=75  GraphicOpacity=smiData.Solid(8).opacity
  Transform : sm_lib/Frames and Transforms/Rigid Transform  TranslationMethod=Cartesian  TranslationStandardOffset=0  TranslationStandardOffsetUnits=m  TranslationStandardAxis=+Z  TranslationCartesianOffset=smiData.RigidTransform(20).translation  TranslationCartesianOffsetUnits=mm  TranslationROffset=0  TranslationROffsetUnits=m  TranslationZOffset=0  TranslationZOffsetUnits=m  TranslationThetaOffset=0  TranslationThetaOffsetUnits=deg  RotationMethod=ArbitraryAxis  RotationAngleUnits=rad  RotationStandardAxis=+Z  RotationAngle=smiData.RigidTransform(20).angle  RotationArbitraryAxis=smiData.RigidTransform(20).axis  FollAlignAxisA=+X  BaseAlignAxisA=+Y  FollAlignAxisB=+Y  BaseAlignAxisB=+Z  RotationSequenceAxes=FollowerAxes  RotationSequence=XYX  RotationSequenceAngles=[0 0 0]  RotationSequenceAnglesUnits=deg  RotationMatrix=[1 0 0; 0 1 0; 0 0 1]  Quaternion=[1 0 0 0]
  F : PMIOPort  Side=Left
  connections:
  ReferenceFrame/RConn1 -- Solid/RConn1 -- Transform/LConn1
  Transform/RConn1 -- F/RConn1

== system Hexa_CAD_ANSFT_Sim_V3/6DoF_Dynamics/APC_8X3_8_Slow_Flyer_2_RIGID ==
  ReferenceFrame : sm_lib/Frames and Transforms/Reference Frame
  Solid : sm_lib/Body Elements/File Solid  ExtGeomFileName=APC 8X3.8 Slow Flyer_Valor predeterminado_sldprt.STEP  UnitType=FromFile  ExtGeomFileUnits=m  StepReaderType=HEX  ExportConvexHullGeometry=off  InertiaType=Custom  Mass=smiData.Solid(8).mass  MassUnits=kg  CenterOfMass=smiData.Solid(8).CoM  CenterOfMassUnits=mm  MomentsOfInertia=smiData.Solid(8).MoI  MomentsOfInertiaUnits=kg*mm^2  ProductsOfInertia=smiData.Solid(8).PoI  ProductsOfInertiaUnits=kg*mm^2  BasedOnType=DensityFromFile  Density=1000  DensityUnits=kg/m^3  DoExposeReferenceFrame=on  SerializedFrames=<Frames/>  GraphicType=FromGeometry  MarkerShape=Sphere  MarkerSize=10  GraphicVisPropType=SimpleVisualProperties  GraphicDiffuseColor=smiData.Solid(8).color  GraphicSpecularColor=[0.5 0.5 0.5 1.0]  GraphicAmbientColor=[0.15 0.15 0.15 1.0]  GraphicEmissiveColor=[0.0 0.0 0.0 1.0]  GraphicShininess=75  GraphicOpacity=smiData.Solid(8).opacity
  Transform : sm_lib/Frames and Transforms/Rigid Transform  TranslationMethod=Cartesian  TranslationStandardOffset=0  TranslationStandardOffsetUnits=m  TranslationStandardAxis=+Z  TranslationCartesianOffset=smiData.RigidTransform(26).translation  TranslationCartesianOffsetUnits=mm  TranslationROffset=0  TranslationROffsetUnits=m  TranslationZOffset=0  TranslationZOffsetUnits=m  TranslationThetaOffset=0  TranslationThetaOffsetUnits=deg  RotationMethod=ArbitraryAxis  RotationAngleUnits=rad  RotationStandardAxis=+Z  RotationAngle=smiData.RigidTransform(26).angle  RotationArbitraryAxis=smiData.RigidTransform(26).axis  FollAlignAxisA=+X  BaseAlignAxisA=+Y  FollAlignAxisB=+Y  BaseAlignAxisB=+Z  RotationSequenceAxes=FollowerAxes  RotationSequence=XYX  RotationSequenceAngles=[0 0 0]  RotationSequenceAnglesUnits=deg  RotationMatrix=[1 0 0; 0 1 0; 0 0 1]  Quaternion=[1 0 0 0]
  F : PMIOPort  Side=Left
  connections:
  ReferenceFrame/RConn1 -- Solid/RConn1 -- Transform/LConn1
  Transform/RConn1 -- F/RConn1

== system Hexa_CAD_ANSFT_Sim_V3/6DoF_Dynamics/APC_8X3_8_Slow_Flyer_3_RIGID ==
  ReferenceFrame : sm_lib/Frames and Transforms/Reference Frame
  Solid : sm_lib/Body Elements/File Solid  ExtGeomFileName=APC 8X3.8 Slow Flyer_Valor predeterminado_sldprt.STEP  UnitType=FromFile  ExtGeomFileUnits=m  StepReaderType=HEX  ExportConvexHullGeometry=off  InertiaType=Custom  Mass=smiData.Solid(8).mass  MassUnits=kg  CenterOfMass=smiData.Solid(8).CoM  CenterOfMassUnits=mm  MomentsOfInertia=smiData.Solid(8).MoI  MomentsOfInertiaUnits=kg*mm^2  ProductsOfInertia=smiData.Solid(8).PoI  ProductsOfInertiaUnits=kg*mm^2  BasedOnType=DensityFromFile  Density=1000  DensityUnits=kg/m^3  DoExposeReferenceFrame=on  SerializedFrames=<Frames/>  GraphicType=FromGeometry  MarkerShape=Sphere  MarkerSize=10  GraphicVisPropType=SimpleVisualProperties  GraphicDiffuseColor=smiData.Solid(8).color  GraphicSpecularColor=[0.5 0.5 0.5 1.0]  GraphicAmbientColor=[0.15 0.15 0.15 1.0]  GraphicEmissiveColor=[0.0 0.0 0.0 1.0]  GraphicShininess=75  GraphicOpacity=smiData.Solid(8).opacity
  Transform : sm_lib/Frames and Transforms/Rigid Transform  TranslationMethod=Cartesian  TranslationStandardOffset=0  TranslationStandardOffsetUnits=m  TranslationStandardAxis=+Z  TranslationCartesianOffset=smiData.RigidTransform(28).translation  TranslationCartesianOffsetUnits=mm  TranslationROffset=0  TranslationROffsetUnits=m  TranslationZOffset=0  TranslationZOffsetUnits=m  TranslationThetaOffset=0  TranslationThetaOffsetUnits=deg  RotationMethod=ArbitraryAxis  RotationAngleUnits=rad  RotationStandardAxis=+Z  RotationAngle=smiData.RigidTransform(28).angle  RotationArbitraryAxis=smiData.RigidTransform(28).axis  FollAlignAxisA=+X  BaseAlignAxisA=+Y  FollAlignAxisB=+Y  BaseAlignAxisB=+Z  RotationSequenceAxes=FollowerAxes  RotationSequence=XYX  RotationSequenceAngles=[0 0 0]  RotationSequenceAnglesUnits=deg  RotationMatrix=[1 0 0; 0 1 0; 0 0 1]  Quaternion=[1 0 0 0]
  F : PMIOPort  Side=Left
  connections:
  ReferenceFrame/RConn1 -- Solid/RConn1 -- Transform/LConn1
  Transform/RConn1 -- F/RConn1

== system Hexa_CAD_ANSFT_Sim_V3/6DoF_Dynamics/APC_8X3_8_Slow_Flyer_4_RIGID ==
  ReferenceFrame : sm_lib/Frames and Transforms/Reference Frame
  Solid : sm_lib/Body Elements/File Solid  ExtGeomFileName=APC 8X3.8 Slow Flyer_Valor predeterminado_sldprt.STEP  UnitType=FromFile  ExtGeomFileUnits=m  StepReaderType=HEX  ExportConvexHullGeometry=off  InertiaType=Custom  Mass=smiData.Solid(8).mass  MassUnits=kg  CenterOfMass=smiData.Solid(8).CoM  CenterOfMassUnits=mm  MomentsOfInertia=smiData.Solid(8).MoI  MomentsOfInertiaUnits=kg*mm^2  ProductsOfInertia=smiData.Solid(8).PoI  ProductsOfInertiaUnits=kg*mm^2  BasedOnType=DensityFromFile  Density=1000  DensityUnits=kg/m^3  DoExposeReferenceFrame=on  SerializedFrames=<Frames/>  GraphicType=FromGeometry  MarkerShape=Sphere  MarkerSize=10  GraphicVisPropType=SimpleVisualProperties  GraphicDiffuseColor=smiData.Solid(8).color  GraphicSpecularColor=[0.5 0.5 0.5 1.0]  GraphicAmbientColor=[0.15 0.15 0.15 1.0]  GraphicEmissiveColor=[0.0 0.0 0.0 1.0]  GraphicShininess=75  GraphicOpacity=smiData.Solid(8).opacity
  Transform : sm_lib/Frames and Transforms/Rigid Transform  TranslationMethod=Cartesian  TranslationStandardOffset=0  TranslationStandardOffsetUnits=m  TranslationStandardAxis=+Z  TranslationCartesianOffset=smiData.RigidTransform(34).translation  TranslationCartesianOffsetUnits=mm  TranslationROffset=0  TranslationROffsetUnits=m  TranslationZOffset=0  TranslationZOffsetUnits=m  TranslationThetaOffset=0  TranslationThetaOffsetUnits=deg  RotationMethod=ArbitraryAxis  RotationAngleUnits=rad  RotationStandardAxis=+Z  RotationAngle=smiData.RigidTransform(34).angle  RotationArbitraryAxis=smiData.RigidTransform(34).axis  FollAlignAxisA=+X  BaseAlignAxisA=+Y  FollAlignAxisB=+Y  BaseAlignAxisB=+Z  RotationSequenceAxes=FollowerAxes  RotationSequence=XYX  RotationSequenceAngles=[0 0 0]  RotationSequenceAnglesUnits=deg  RotationMatrix=[1 0 0; 0 1 0; 0 0 1]  Quaternion=[1 0 0 0]
  F : PMIOPort  Side=Left
  connections:
  ReferenceFrame/RConn1 -- Solid/RConn1 -- Transform/LConn1
  Transform/RConn1 -- F/RConn1

== system Hexa_CAD_ANSFT_Sim_V3/6DoF_Dynamics/APC_8X3_8_Slow_Flyer_5_RIGID ==
  ReferenceFrame : sm_lib/Frames and Transforms/Reference Frame
  Solid : sm_lib/Body Elements/File Solid  ExtGeomFileName=APC 8X3.8 Slow Flyer_Valor predeterminado_sldprt.STEP  UnitType=FromFile  ExtGeomFileUnits=m  StepReaderType=HEX  ExportConvexHullGeometry=off  InertiaType=Custom  Mass=smiData.Solid(8).mass  MassUnits=kg  CenterOfMass=smiData.Solid(8).CoM  CenterOfMassUnits=mm  MomentsOfInertia=smiData.Solid(8).MoI  MomentsOfInertiaUnits=kg*mm^2  ProductsOfInertia=smiData.Solid(8).PoI  ProductsOfInertiaUnits=kg*mm^2  BasedOnType=DensityFromFile  Density=1000  DensityUnits=kg/m^3  DoExposeReferenceFrame=on  SerializedFrames=<Frames/>  GraphicType=FromGeometry  MarkerShape=Sphere  MarkerSize=10  GraphicVisPropType=SimpleVisualProperties  GraphicDiffuseColor=smiData.Solid(8).color  GraphicSpecularColor=[0.5 0.5 0.5 1.0]  GraphicAmbientColor=[0.15 0.15 0.15 1.0]  GraphicEmissiveColor=[0.0 0.0 0.0 1.0]  GraphicShininess=75  GraphicOpacity=smiData.Solid(8).opacity
  Transform : sm_lib/Frames and Transforms/Rigid Transform  TranslationMethod=Cartesian  TranslationStandardOffset=0  TranslationStandardOffsetUnits=m  TranslationStandardAxis=+Z  TranslationCartesianOffset=smiData.RigidTransform(36).translation  TranslationCartesianOffsetUnits=mm  TranslationROffset=0  TranslationROffsetUnits=m  TranslationZOffset=0  TranslationZOffsetUnits=m  TranslationThetaOffset=0  TranslationThetaOffsetUnits=deg  RotationMethod=ArbitraryAxis  RotationAngleUnits=rad  RotationStandardAxis=+Z  RotationAngle=smiData.RigidTransform(36).angle  RotationArbitraryAxis=smiData.RigidTransform(36).axis  FollAlignAxisA=+X  BaseAlignAxisA=+Y  FollAlignAxisB=+Y  BaseAlignAxisB=+Z  RotationSequenceAxes=FollowerAxes  RotationSequence=XYX  RotationSequenceAngles=[0 0 0]  RotationSequenceAnglesUnits=deg  RotationMatrix=[1 0 0; 0 1 0; 0 0 1]  Quaternion=[1 0 0 0]
  F : PMIOPort  Side=Left
  connections:
  ReferenceFrame/RConn1 -- Solid/RConn1 -- Transform/LConn1
  Transform/RConn1 -- F/RConn1

== system Hexa_CAD_ANSFT_Sim_V3/6DoF_Dynamics/APC_8X3_8_Slow_Flyer_6_RIGID ==
  ReferenceFrame : sm_lib/Frames and Transforms/Reference Frame
  Solid : sm_lib/Body Elements/File Solid  ExtGeomFileName=APC 8X3.8 Slow Flyer_Valor predeterminado_sldprt.STEP  UnitType=FromFile  ExtGeomFileUnits=m  StepReaderType=HEX  ExportConvexHullGeometry=off  InertiaType=Custom  Mass=smiData.Solid(8).mass  MassUnits=kg  CenterOfMass=smiData.Solid(8).CoM  CenterOfMassUnits=mm  MomentsOfInertia=smiData.Solid(8).MoI  MomentsOfInertiaUnits=kg*mm^2  ProductsOfInertia=smiData.Solid(8).PoI  ProductsOfInertiaUnits=kg*mm^2  BasedOnType=DensityFromFile  Density=1000  DensityUnits=kg/m^3  DoExposeReferenceFrame=on  SerializedFrames=<Frames/>  GraphicType=FromGeometry  MarkerShape=Sphere  MarkerSize=10  GraphicVisPropType=SimpleVisualProperties  GraphicDiffuseColor=smiData.Solid(8).color  GraphicSpecularColor=[0.5 0.5 0.5 1.0]  GraphicAmbientColor=[0.15 0.15 0.15 1.0]  GraphicEmissiveColor=[0.0 0.0 0.0 1.0]  GraphicShininess=75  GraphicOpacity=smiData.Solid(8).opacity
  Transform : sm_lib/Frames and Transforms/Rigid Transform  TranslationMethod=Cartesian  TranslationStandardOffset=0  TranslationStandardOffsetUnits=m  TranslationStandardAxis=+Z  TranslationCartesianOffset=smiData.RigidTransform(42).translation  TranslationCartesianOffsetUnits=mm  TranslationROffset=0  TranslationROffsetUnits=m  TranslationZOffset=0  TranslationZOffsetUnits=m  TranslationThetaOffset=0  TranslationThetaOffsetUnits=deg  RotationMethod=ArbitraryAxis  RotationAngleUnits=rad  RotationStandardAxis=+Z  RotationAngle=smiData.RigidTransform(42).angle  RotationArbitraryAxis=smiData.RigidTransform(42).axis  FollAlignAxisA=+X  BaseAlignAxisA=+Y  FollAlignAxisB=+Y  BaseAlignAxisB=+Z  RotationSequenceAxes=FollowerAxes  RotationSequence=XYX  RotationSequenceAngles=[0 0 0]  RotationSequenceAnglesUnits=deg  RotationMatrix=[1 0 0; 0 1 0; 0 0 1]  Quaternion=[1 0 0 0]
  F : PMIOPort  Side=Left
  connections:
  ReferenceFrame/RConn1 -- Solid/RConn1 -- Transform/LConn1
  Transform/RConn1 -- F/RConn1

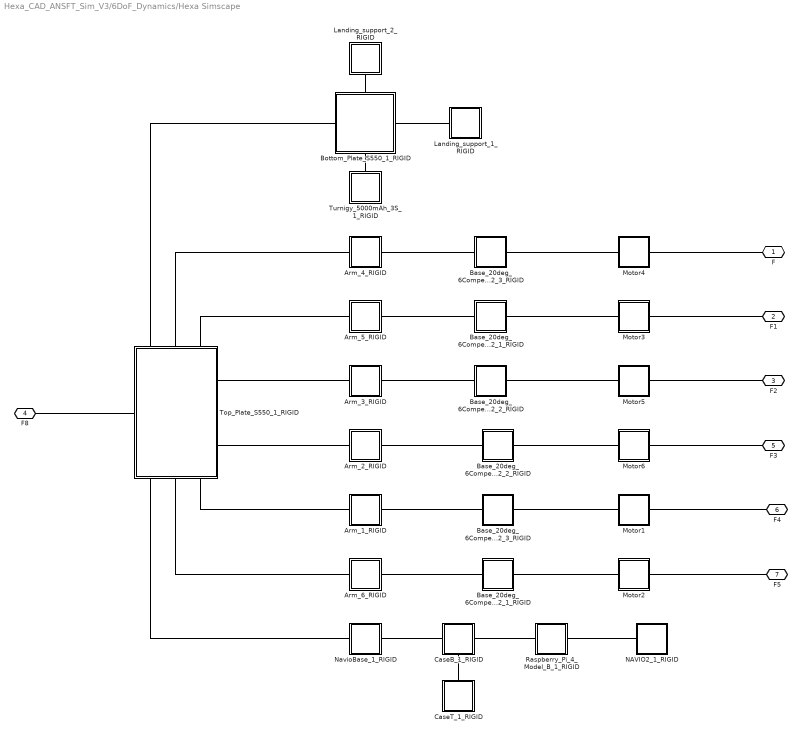
== system Hexa_CAD_ANSFT_Sim_V3/6DoF_Dynamics/Hexa Simscape ==
  Arm_1_RIGID : Subsystem
  Arm_2_RIGID : Subsystem
  Arm_3_RIGID : Subsystem
  Arm_4_RIGID : Subsystem
  Arm_5_RIGID : Subsystem
  Arm_6_RIGID : Subsystem
  Base_20deg_6Compensation_Motor1_3_5_V2_1_RIGID : Subsystem
  Base_20deg_6Compensation_Motor1_3_5_V2_2_RIGID : Subsystem
  Base_20deg_6Compensation_Motor1_3_5_V2_3_RIGID : Subsystem
  Base_20deg_6Compensation_Motor2_4_6_V2_1_RIGID : Subsystem
  Base_20deg_6Compensation_Motor2_4_6_V2_2_RIGID : Subsystem
  Base_20deg_6Compensation_Motor2_4_6_V2_3_RIGID : Subsystem
  Bottom_Plate_S550_1_RIGID : Subsystem
      settings: PortSchema="{\"entries\":[{\"content\":{\"sides\":[{\"content\":{\"connectorIds\":[\"LConn1\"]},\"type\":\"ConnectorPlacement.EquallySpacedRectSide\",\"uuid\":\"b60aee1b-46ea-46f0-a05c-bf417081e61d\"},{\"content\":{\"connectorIds\":[\"RConn1\"],\"side\":\"RIGHT\"},\"type\":\"ConnectorPlacement.EquallySpacedRectSide\",\"uuid\":\"cd97571d-2e2b-4347-9b07-d71076a84794\"},{\"content\":{\"connectorIds\":[\"LConn2\"],\"side\":\"TOP\"},\"type\":\"ConnectorPlacement.EquallySpacedRectSide\",\"uuid\":\"bbcac78d-4cfc-4b87-aefa-5145f856d219\"},{\"content\":{\"connectorIds\":[\"RConn2\"],\"side\":\"BOTTOM\"},\"type\":\"ConnectorPlacement.EquallySpacedRectSide\",\"uuid\":\"65d48ba4-c897-4101-9e53-f004230c2534\"}]},\"type\":\"ConnectorPlacement.EquallySpacedConnector\",\"uuid\":\"4e9dcdc4-a5dc-425d-ae78-89d2a265ea75\"}],\"packageUris\":[\"http://schema.mathworks.com/mf0/Connector/R2020b\"],\"version\":\"1.0\"}"
  CaseB_1_RIGID : Subsystem
      settings: PortSchema="{\"entries\":[{\"content\":{\"sides\":[{\"content\":{\"connectorIds\":[\"LConn1\"]},\"type\":\"ConnectorPlacement.EquallySpacedRectSide\",\"uuid\":\"e0e2ffdf-f4b4-41c8-99a3-2acb5eae189e\"},{\"content\":{\"connectorIds\":[\"RConn1\"],\"side\":\"RIGHT\"},\"type\":\"ConnectorPlacement.EquallySpacedRectSide\",\"uuid\":\"05d64d9d-d627-4e31-8e39-4fab0a50d960\"},{\"content\":{\"side\":\"TOP\"},\"type\":\"ConnectorPlacement.EquallySpacedRectSide\",\"uuid\":\"4ff7e761-be68-4dd2-8dc5-84f74b883614\"},{\"content\":{\"connectorIds\":[\"RConn2\"],\"side\":\"BOTTOM\"},\"type\":\"ConnectorPlacement.EquallySpacedRectSide\",\"uuid\":\"3a36ff3a-ee2e-4c24-8945-c869eb2d25b3\"}]},\"type\":\"ConnectorPlacement.EquallySpacedConnector\",\"uuid\":\"dbcbf738-7f4d-496b-b6b7-830c52fa5dc5\"}],\"packageUris\":[\"http://schema.mathworks.com/mf0/Connector/R2020b\"],\"version\":\"1.0\"}"
  CaseT_1_RIGID : Subsystem
      settings: PortSchema="{\"entries\":[{\"content\":{\"sides\":[{\"content\":{},\"type\":\"ConnectorPlacement.EquallySpacedRectSide\",\"uuid\":\"576ac322-0dfb-4909-87c2-bf8a263a358e\"},{\"content\":{\"side\":\"RIGHT\"},\"type\":\"ConnectorPlacement.EquallySpacedRectSide\",\"uuid\":\"5e414c09-2810-44ec-9656-6c32e1f740f3\"},{\"content\":{\"connectorIds\":[\"LConn1\"],\"side\":\"TOP\"},\"type\":\"ConnectorPlacement.EquallySpacedRectSide\",\"uuid\":\"25f18d4e-8b9a-4e2a-b77b-73719c542d66\"},{\"content\":{\"side\":\"BOTTOM\"},\"type\":\"ConnectorPlacement.EquallySpacedRectSide\",\"uuid\":\"17e7d79d-6e5a-4285-9e4e-54d9f62b24d7\"}]},\"type\":\"ConnectorPlacement.EquallySpacedConnector\",\"uuid\":\"763568b0-0d5c-494d-b330-ee4b036660ee\"}],\"packageUris\":[\"http://schema.mathworks.com/mf0/Connector/R2020b\"],\"version\":\"1.0\"}"
  Landing_support_1_RIGID : Subsystem
  Landing_support_2_RIGID : Subsystem
      settings: PortSchema="{\"entries\":[{\"content\":{\"sides\":[{\"content\":{},\"type\":\"ConnectorPlacement.EquallySpacedRectSide\",\"uuid\":\"576ac322-0dfb-4909-87c2-bf8a263a358e\"},{\"content\":{\"side\":\"RIGHT\"},\"type\":\"ConnectorPlacement.EquallySpacedRectSide\",\"uuid\":\"5e414c09-2810-44ec-9656-6c32e1f740f3\"},{\"content\":{\"side\":\"TOP\"},\"type\":\"ConnectorPlacement.EquallySpacedRectSide\",\"uuid\":\"25f18d4e-8b9a-4e2a-b77b-73719c542d66\"},{\"content\":{\"connectorIds\":[\"RConn1\"],\"side\":\"BOTTOM\"},\"type\":\"ConnectorPlacement.EquallySpacedRectSide\",\"uuid\":\"2ec4f2a5-39d2-4589-98f3-94078b0eb089\"}]},\"type\":\"ConnectorPlacement.EquallySpacedConnector\",\"uuid\":\"763568b0-0d5c-494d-b330-ee4b036660ee\"}],\"packageUris\":[\"http://schema.mathworks.com/mf0/Connector/R2020b\"],\"version\":\"1.0\"}"
  Motor1 : Subsystem
  Motor2 : Subsystem
  Motor3 : Subsystem
  Motor4 : Subsystem
  Motor5 : Subsystem
  Motor6 : Subsystem
  NAVIO2_1_RIGID : Subsystem
  NavioBase_1_RIGID : Subsystem
  Raspberry_Pi_4_Model_B_1_RIGID : Subsystem
  Top_Plate_S550_1_RIGID : Subsystem
      settings: PortSchema="{\"entries\":[{\"content\":{\"sides\":[{\"content\":{\"connectorIds\":[\"LConn1\"]},\"type\":\"ConnectorPlacement.EquallySpacedRectSide\",\"uuid\":\"38be4f7c-e8f0-45bd-aaae-e8e225420879\"},{\"content\":{\"connectorIds\":[\"RConn1\",\"RConn2\"],\"side\":\"RIGHT\"},\"type\":\"ConnectorPlacement.EquallySpacedRectSide\",\"uuid\":\"643fb6d5-793f-449a-be28-dc16e548e0f0\"},{\"content\":{\"connectorIds\":[\"LConn2\",\"LConn3\",\"LConn4\"],\"side\":\"TOP\"},\"type\":\"ConnectorPlacement.EquallySpacedRectSide\",\"uuid\":\"b49d8ad6-4208-4be1-be14-726d46acfdf9\"},{\"content\":{\"connectorIds\":[\"RConn3\",\"RConn4\",\"RConn5\"],\"side\":\"BOTTOM\"},\"type\":\"ConnectorPlacement.EquallySpacedRectSide\",\"uuid\":\"d7cfdf48-def5-424f-b9db-91b08a499752\"}]},\"type\":\"ConnectorPlacement.EquallySpacedConnector\",\"uuid\":\"f674dc6c-c053-4b4e-b3eb-09a53e21b2b3\"}],\"packageUris\":[\"http://schema.mathworks.com/mf0/Connector/R2020b\"],\"version\":\"1.0\"}"
  Turnigy_5000mAh_3S_1_RIGID : Subsystem
      settings: PortSchema="{\"entries\":[{\"content\":{\"sides\":[{\"content\":{},\"type\":\"ConnectorPlacement.EquallySpacedRectSide\",\"uuid\":\"576ac322-0dfb-4909-87c2-bf8a263a358e\"},{\"content\":{\"side\":\"RIGHT\"},\"type\":\"ConnectorPlacement.EquallySpacedRectSide\",\"uuid\":\"5e414c09-2810-44ec-9656-6c32e1f740f3\"},{\"content\":{\"connectorIds\":[\"LConn1\"],\"side\":\"TOP\"},\"type\":\"ConnectorPlacement.EquallySpacedRectSide\",\"uuid\":\"25f18d4e-8b9a-4e2a-b77b-73719c542d66\"}]},\"type\":\"ConnectorPlacement.EquallySpacedConnector\",\"uuid\":\"763568b0-0d5c-494d-b330-ee4b036660ee\"}],\"packageUris\":[\"http://schema.mathworks.com/mf0/Connector/R2020b\"],\"version\":\"1.0\"}"
  F : PMIOPort  Side=Right
  F1 : PMIOPort  Port=2  Side=Right
  F2 : PMIOPort  Port=3  Side=Right
  F8 : PMIOPort  Port=4  Side=Left
  F3 : PMIOPort  Port=5  Side=Right
  F4 : PMIOPort  Port=6  Side=Right
  F5 : PMIOPort  Port=7  Side=Right
  connections:
  Motor3/LConn1 -- Base_20deg_6Compensation_Motor2_4_6_V2_1_RIGID/RConn1
  Motor4/LConn1 -- Base_20deg_6Compensation_Motor1_3_5_V2_3_RIGID/RConn1
  Motor5/LConn1 -- Base_20deg_6Compensation_Motor2_4_6_V2_2_RIGID/RConn1
  Arm_1_RIGID/RConn1 -- Base_20deg_6Compensation_Motor2_4_6_V2_3_RIGID/LConn1
  Motor2/LConn1 -- Base_20deg_6Compensation_Motor1_3_5_V2_1_RIGID/RConn1
  NavioBase_1_RIGID/LConn1 -- Top_Plate_S550_1_RIGID/RConn3
  NAVIO2_1_RIGID/LConn1 -- Raspberry_Pi_4_Model_B_1_RIGID/RConn1
  CaseB_1_RIGID/LConn1 -- NavioBase_1_RIGID/RConn1
  Motor6/RConn1 -- F3/RConn1
  Bottom_Plate_S550_1_RIGID/RConn2 -- Turnigy_5000mAh_3S_1_RIGID/LConn1
  CaseB_1_RIGID/RConn1 -- Raspberry_Pi_4_Model_B_1_RIGID/LConn1
  Arm_1_RIGID/LConn1 -- Top_Plate_S550_1_RIGID/RConn5
  Arm_5_RIGID/RConn1 -- Base_20deg_6Compensation_Motor2_4_6_V2_1_RIGID/LConn1
  Bottom_Plate_S550_1_RIGID/RConn1 -- Landing_support_1_RIGID/LConn1
  Motor6/LConn1 -- Base_20deg_6Compensation_Motor1_3_5_V2_2_RIGID/RConn1
  Arm_6_RIGID/RConn1 -- Base_20deg_6Compensation_Motor1_3_5_V2_1_RIGID/LConn1
  CaseB_1_RIGID/RConn2 -- CaseT_1_RIGID/LConn1
  Top_Plate_S550_1_RIGID/LConn1 -- F8/RConn1
  Arm_3_RIGID/LConn1 -- Top_Plate_S550_1_RIGID/RConn1
  Arm_6_RIGID/LConn1 -- Top_Plate_S550_1_RIGID/RConn4
  Arm_2_RIGID/RConn1 -- Base_20deg_6Compensation_Motor1_3_5_V2_2_RIGID/LConn1
  Arm_4_RIGID/RConn1 -- Base_20deg_6Compensation_Motor1_3_5_V2_3_RIGID/LConn1
  Motor1/RConn1 -- F4/RConn1
  Arm_3_RIGID/RConn1 -- Base_20deg_6Compensation_Motor2_4_6_V2_2_RIGID/LConn1
  Arm_4_RIGID/LConn1 -- Top_Plate_S550_1_RIGID/LConn3
  Arm_5_RIGID/LConn1 -- Top_Plate_S550_1_RIGID/LConn4
  Motor2/RConn1 -- F5/RConn1
  Bottom_Plate_S550_1_RIGID/LConn1 -- Top_Plate_S550_1_RIGID/LConn2
  Bottom_Plate_S550_1_RIGID/LConn2 -- Landing_support_2_RIGID/RConn1
  Arm_2_RIGID/LConn1 -- Top_Plate_S550_1_RIGID/RConn2
  Motor1/LConn1 -- Base_20deg_6Compensation_Motor2_4_6_V2_3_RIGID/RConn1
  Motor5/RConn1 -- F2/RConn1
  Motor3/RConn1 -- F1/RConn1
  Motor4/RConn1 -- F/RConn1
